simulink model "prob7_sub"  (R2020a)
settings: Solver=FixedStepAuto  StartTime=0.0  StopTime=10.0  FixedStep=0.2  RelTol=1e-3
settings Model: Creator='Z'ome  LastModifiedBy='Z'ome
settings DataIOCC: SaveOutput=off  SaveTime=off

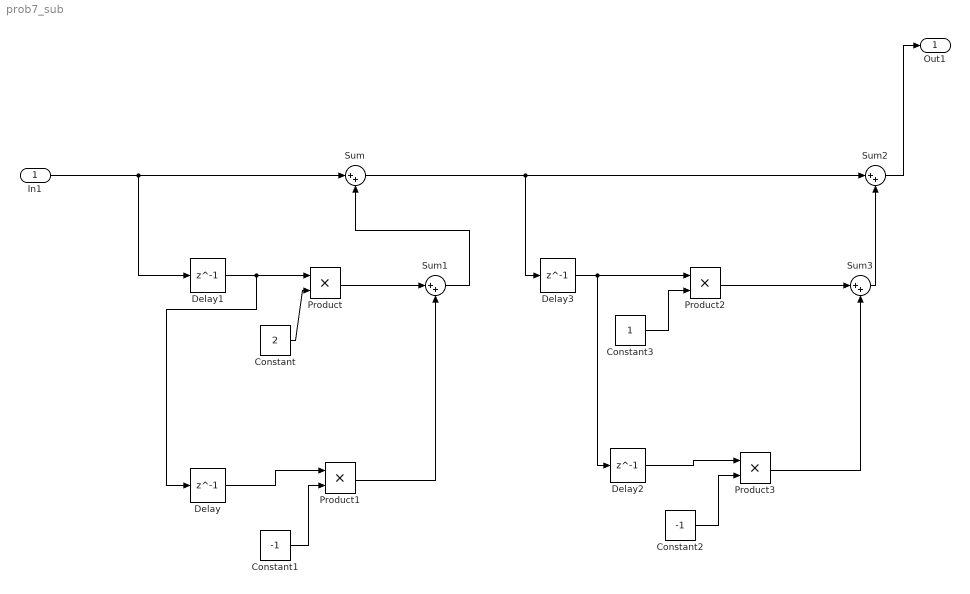
== system prob7_sub ==
  In1 : Inport  OutDataTypeStr=double  PortDimensions=1  SampleTime=[0.20000000000000001,0]
  Constant : Constant  Value=2
  Constant1 : Constant  Value=-1
  Constant2 : Constant  Value=-1
  Constant3 : Constant
  Delay{,1..3} (4 alike) : Delay  DelayLength=1
  Product{,1..3} (4 alike) : Product
  Sum{,1..3} (4 alike) : Sum  Inputs=|++
  Out1 : Outport  OutDataTypeStr=double  PortDimensions=1  SampleTime=[0.20000000000000001,0]
  wires:
  Constant3/1 -> Product2/2
  Delay2/1 -> Product3/1
  Delay3/1 -> Product2/1, Delay2/1
  In1/1 -> Sum/1, Delay1/1
  Sum3/1 -> Sum2/2
  Product1/1 -> Sum1/2
  Constant2/1 -> Product3/2
  Product/1 -> Sum1/1
  Constant/1 -> Product/2
  Sum/1 -> Sum2/1, Delay3/1
  Constant1/1 -> Product1/2
  Product2/1 -> Sum3/1
  Delay/1 -> Product1/1
  Product3/1 -> Sum3/2
  Delay1/1 -> Product/1, Delay/1
  Sum1/1 -> Sum/2
  Sum2/1 -> Out1/1
